simulink model "controladorNovo"  (R2018a)
settings: Solver=FixedStepDiscrete  StartTime=0.0  StopTime=tmax  FixedStep=h  RelTol=1e-3
values from neighbouring files (symbols this model uses):
  h = 0.01    [init.m]    (also in initTemp.m)
  x0 = [1;1]    [init.m]
undefined symbols (not defined in the file or in its folder): Cd, gama, H, phi
libraries: dspsrcs4 x2, simulink x1
settings Model: Creator=Raposo  LastModifiedBy=raposo
settings OptimizationCC: LifeSpan=inf
settings DebuggingCC: AllowSymbolicDim=off  SFExecutionAtInitializationDiag=none
settings HardwareCC: ProdBitPerSizeT=32  ProdBitPerPtrDiffT=32  ProdWordSize=32  ProdHWDeviceType=Specified
settings CodeAppCC: StateflowObjectComments=on

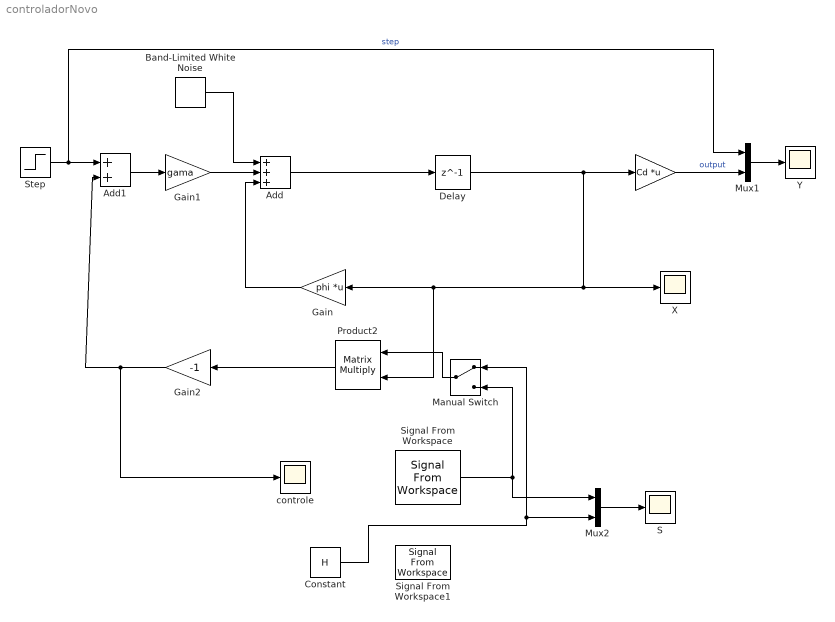
== system controladorNovo ==
  " " : Gain  Gain=Cd  Multiplication=Matrix(K*u)
  Add : Sum  Inputs=+++
  Add1 : Sum
  Band-Limited White Noise : simulink/Sources/Band-Limited White Noise  Cov=[0.00000001]*0  Ts=h  seed=[23341]
  Constant : Constant  Value=H  VectorParams1D=off
  Delay : Delay  DelayLength=1  InitialCondition=x0  SampleTime=h
  Gain : Gain  Gain=phi  Multiplication=Matrix(K*u)
  Gain1 : Gain  Gain=gama
  Gain2 : Gain  Gain=-1
  Manual Switch : ManualSwitch
  Mux1 : Mux  Inputs=2
  Mux2 : Mux  Inputs=2
  Product2 : Product  Multiplication=Matrix(*)
  S : Scope
  Signal From Workspace : dspsrcs4/Signal From Workspace  X=lx'  Ts=1  nsamps=1  OutputAfterFinalValue=Setting to zero  ignoreOrWarnInputAndFrameLengths=off  OutputFrames=on
  Signal From Workspace1 : dspsrcs4/Signal From Workspace  X=H  Ts=h  nsamps=1  OutputAfterFinalValue=Setting to zero  ignoreOrWarnInputAndFrameLengths=off  OutputFrames=on
  Step : Step  After=0  SampleTime=h
  X : Scope
  Y : Scope
  controle : Scope
  wires:
  Band-Limited White Noise/1 -> Add/1
  Gain/1 -> Add/3
  Delay/1 -> X/1, Product2/2, Gain/1, " "/1
  Signal From Workspace/1 -> Manual Switch/2, Mux2/1
  Step/1 -> Mux1/1, Add1/1  "step"
  Mux1/1 -> Y/1
  " "/1 -> Mux1/2  "output"
  Mux2/1 -> S/1
  Add1/1 -> Gain1/1
  Gain1/1 -> Add/2
  Add/1 -> Delay/1
  Product2/1 -> Gain2/1
  Gain2/1 -> controle/1, Add1/2
  Constant/1 -> Mux2/2, Manual Switch/1
  Manual Switch/1 -> Product2/1
